simulink model "Rearranged_With_Subsystems"  (R2022b)
settings: Solver=ode15s  StartTime=0.0  StopTime=400  RelTol=1e-3
InitFcn:
  | ManipulatorSetup
  | init_quad_new_leg_raibert_strategy_v2
values from neighbouring files (symbols this model uses):
  body = 'obstacle'+string(i)    [GUIWithNavigation.m]    (also in RunModel.m)
  endx = 18    [EnvironmentData.mat]    (also in Practice data.mat = 15)
  endy = 18    [EnvironmentData.mat]    (also in Practice data.mat = 14)
  floorl = 20    [EnvironmentData.mat]    (also in GUIWithNavigation.m; Practice data.mat; RunModel.m)
  floorw = 20    [EnvironmentData.mat]    (also in GUIWithNavigation.m; Practice data.mat; RunModel.m)
  planner = plannerRRTStar(ss,stateValidator)    [GUIWithNavigation.m]    (also in RunModel.m)
  startx = 3    [EnvironmentData.mat]    (also in Practice data.mat = 2)
  starty = 3    [EnvironmentData.mat]    (also in Practice data.mat = 2)
  tar1Len = 10    [EnvironmentData.mat]    (also in GUIWithNavigation.m = length(target1); Practice data.mat = 13; RunModel.m = length(target1))
  target = [3 4.99844642156 6.95141646815 8.78790598722 9.67257563911 9.70990834754 10.5092252376 9.30187214417 9.05327436398 9.4 9.4 10.8486938703 ... (44 elements, 22x2)]    [EnvironmentData.mat]    (also in GUIWithNavigation.m = cat(1,target1,target2); Practice data.mat = [2 3.44057581018 5.07942513831 5.42542290116 7.21306818311 8; RunModel.m = cat(1,target1,target2))
  tarLen = 22    [EnvironmentData.mat]    (also in RunModel.m = length(target))
undefined symbols (not defined in the file or in its folder): closeFingers, ctrl, Extr_Data_LinkEndHole, grabObjectAngles, grabObjectAngles2, ground, holdFingers, homeAngles, inverseKinematicWeights, l1, l2, m1, m2, openFingers, readyAngles, X, Y, Z
libraries: sm_lib x459, nesl_utility x134, slpidlib x31, fl_ps_legacy_lib x6, robotmaniplib x6, simulink x5, fl_lib x5, Contact_Forces_Lib x4, Parts_Lib x4, sharedtransform x2, dspstat3 x1
(part 15 of 16)

== system Rearranged_With_Subsystems/Quadruped/leg_rr/s_joint_ctrl  ==
  tgt_angle : Inport
  has_ctrl : Inport  Port=2
  PID Controller : slpidlib/PID Controller  Controller=PID  Form=Parallel  TimeDomain=Continuous-time  UseExternalTs=off  SampleTime=-1  IntegratorMethod=Forward Euler  FilterMethod=Forward Euler  ControllerParametersSource=internal  P=ctrl.pos_kp  I=ctrl.pos_ki  UseKiTs=off  D=ctrl.pos_kd  N=100  UseFilter=on  TunerSelectOption=Transfer Function Based (PID Tuner App)  InitialConditionSource=internal  InitialConditionForIntegrator=0  InitialConditionForFilter=0  DifferentiatorICPrevScaledInput=0  ExternalReset=none  TrackingMode=off  Kt=1  LimitOutput=off  SatLimitsSource=internal  UpperSaturationLimit=inf  LowerSaturationLimit=-inf  LinearizeAsGain=on  AntiWindupMode=none  Kb=1  LimitIntegrator=off  UpperIntegratorSaturationLimit=inf  LowerIntegratorSaturationLimit=-inf  POutMin=[]  POutMax=[]  IOutMin=[]  IOutMax=[]  DOutMin=[]  DOutMax=[]  NOutMin=[]  NOutMax=[]  SumOutMin=[]  SumOutMax=[]  SaturationOutMin=[]  SaturationOutMax=[]  PParamMin=[]  PParamMax=[]  IParamMin=[]  IParamMax=[]  DParamMin=[]  DParamMax=[]  NParamMin=[]  NParamMax=[]  KbParamMin=[]  KbParamMax=[]  KtParamMin=[]  KtParamMax=[]  KbOutMin=[]  KbOutMax=[]  KtOutMin=[]  KtOutMax=[]  IntegratorOutMin=[]  IntegratorOutMax=[]  FilterOutMin=[]  FilterOutMax=[]  SumI1OutMin=[]  SumI1OutMax=[]  SumI2OutMin=[]  SumI2OutMax=[]  SumI3OutMin=[]  SumI3OutMax=[]  SumI4OutMin=[]  SumI4OutMax=[]  SumDOutMin=[]  SumDOutMax=[]  DifferentiatorOutMin=[]  DifferentiatorOutMax=[]  FilterDiffOutCoefMin=[]  FilterDiffOutCoefMax=[]  ReciprocalOutMin=[]  ReciprocalOutMax=[]  SumDenOutMin=[]  SumDenOutMax=[]  SumNumOutMin=[]  SumNumOutMax=[]  DivideOutMin=[]  DivideOutMax=[]  UdiffTsProdOutMin=[]  UdiffTsProdOutMax=[]  NTsProdOutMin=[]  NTsProdOutMax=[]  UintegralTsProdOutMin=[]  UintegralTsProdOutMax=[]  UngainTsProdOutMin=[]  UngainTsProdOutMax=[]  ClampingZeroOutDataTypeStr=Inherit: Inherit via back propagation  ClampingZeroOutMin=[]  ClampingZeroOutMax=[]  FilterDenConstantOutDataTypeStr=Inherit: Inherit via back propagation  FilterDenConstantOutMin=[]  FilterDenConstantOutMax=[]  PCopyOutDataTypeStr=Inherit: Inherit via back propagation  PCopyOutMin=[]  PCopyOutMax=[]  NCopyOutDataTypeStr=Inherit: Inherit via back propagation  NCopyOutMin=[]  NCopyOutMax=[]  IntegratorContinuousStateAttributes=''  IntegratorStateMustResolveToSignalObject=off  IntegratorRTWStateStorageClass=Auto  FilterContinuousStateAttributes=''  FilterStateMustResolveToSignalObject=off  FilterRTWStateStorageClass=Auto  ParallelPVariant=InternalParameters  IdealPVariant=Disabled  IVariant=InternalParameters  DVariant=InternalParameters  IntegratorVariant=Continuous  SatVariant=Disabled  AWVariant=Passthrough  PCopyVariant=Disabled  TRVariant=Disabled  FdbkBlocksVariant=Forward  IdealPFdbkVariant=Disabled  SatFdbkVariant=Disabled  DerivativeFilterVariant=ContFilter  NVariant=InternalParameters  NCopyVariant=Disabled  FilterICVariant=InternalICsFilter  IntegratorICVariant=InternalICs  ExternalResetVariant=Disabled  TRSumVariant=Passthrough  SumFdbkVariant=Disabled  SumVariant=Sum_PID  TsampFilterVariant=InternalTs  TsampNgainVariant=Passthrough  TsampIntegralVariant=Passthrough  ExternalSaturationOutDataTypeStr=Inherit: Same as second input
  PID Controller3 : slpidlib/PID Controller  Controller=PID  Form=Parallel  TimeDomain=Continuous-time  UseExternalTs=off  SampleTime=-1  IntegratorMethod=Forward Euler  FilterMethod=Forward Euler  ControllerParametersSource=internal  P=ctrl.vel_kp  I=ctrl.vel_ki  UseKiTs=off  D=ctrl.vel_kd  N=100  UseFilter=on  TunerSelectOption=Transfer Function Based (PID Tuner App)  InitialConditionSource=internal  InitialConditionForIntegrator=0  InitialConditionForFilter=0  DifferentiatorICPrevScaledInput=0  ExternalReset=none  TrackingMode=off  Kt=1  LimitOutput=off  SatLimitsSource=internal  UpperSaturationLimit=inf  LowerSaturationLimit=-inf  LinearizeAsGain=on  AntiWindupMode=none  Kb=1  LimitIntegrator=off  UpperIntegratorSaturationLimit=inf  LowerIntegratorSaturationLimit=-inf  POutMin=[]  POutMax=[]  IOutMin=[]  IOutMax=[]  DOutMin=[]  DOutMax=[]  NOutMin=[]  NOutMax=[]  SumOutMin=[]  SumOutMax=[]  SaturationOutMin=[]  SaturationOutMax=[]  PParamMin=[]  PParamMax=[]  IParamMin=[]  IParamMax=[]  DParamMin=[]  DParamMax=[]  NParamMin=[]  NParamMax=[]  KbParamMin=[]  KbParamMax=[]  KtParamMin=[]  KtParamMax=[]  KbOutMin=[]  KbOutMax=[]  KtOutMin=[]  KtOutMax=[]  IntegratorOutMin=[]  IntegratorOutMax=[]  FilterOutMin=[]  FilterOutMax=[]  SumI1OutMin=[]  SumI1OutMax=[]  SumI2OutMin=[]  SumI2OutMax=[]  SumI3OutMin=[]  SumI3OutMax=[]  SumI4OutMin=[]  SumI4OutMax=[]  SumDOutMin=[]  SumDOutMax=[]  DifferentiatorOutMin=[]  DifferentiatorOutMax=[]  FilterDiffOutCoefMin=[]  FilterDiffOutCoefMax=[]  ReciprocalOutMin=[]  ReciprocalOutMax=[]  SumDenOutMin=[]  SumDenOutMax=[]  SumNumOutMin=[]  SumNumOutMax=[]  DivideOutMin=[]  DivideOutMax=[]  UdiffTsProdOutMin=[]  UdiffTsProdOutMax=[]  NTsProdOutMin=[]  NTsProdOutMax=[]  UintegralTsProdOutMin=[]  UintegralTsProdOutMax=[]  UngainTsProdOutMin=[]  UngainTsProdOutMax=[]  ClampingZeroOutDataTypeStr=Inherit: Inherit via back propagation  ClampingZeroOutMin=[]  ClampingZeroOutMax=[]  FilterDenConstantOutDataTypeStr=Inherit: Inherit via back propagation  FilterDenConstantOutMin=[]  FilterDenConstantOutMax=[]  PCopyOutDataTypeStr=Inherit: Inherit via back propagation  PCopyOutMin=[]  PCopyOutMax=[]  NCopyOutDataTypeStr=Inherit: Inherit via back propagation  NCopyOutMin=[]  NCopyOutMax=[]  IntegratorContinuousStateAttributes=''  IntegratorStateMustResolveToSignalObject=off  IntegratorRTWStateStorageClass=Auto  FilterContinuousStateAttributes=''  FilterStateMustResolveToSignalObject=off  FilterRTWStateStorageClass=Auto  ParallelPVariant=InternalParameters  IdealPVariant=Disabled  IVariant=InternalParameters  DVariant=InternalParameters  IntegratorVariant=Continuous  SatVariant=Disabled  AWVariant=Passthrough  PCopyVariant=Disabled  TRVariant=Disabled  FdbkBlocksVariant=Forward  IdealPFdbkVariant=Disabled  SatFdbkVariant=Disabled  DerivativeFilterVariant=ContFilter  NVariant=InternalParameters  NCopyVariant=Disabled  FilterICVariant=InternalICsFilter  IntegratorICVariant=InternalICs  ExternalResetVariant=Disabled  TRSumVariant=Passthrough  SumFdbkVariant=Disabled  SumVariant=Sum_PID  TsampFilterVariant=InternalTs  TsampNgainVariant=Passthrough  TsampIntegralVariant=Passthrough  ExternalSaturationOutDataTypeStr=Inherit: Same as second input
  PSConv3 : nesl_utility/PS-Simulink Converter  PhysicalDomain=network_engine_domain  SubClassName=ps_output  LeftPortType=input  RightPortType=output  PseudoPeriodic=off  Frequencies=[]  VectorFormat=1-D array  Unit=1  AffineConversion=off
  PSConv4 : nesl_utility/PS-Simulink Converter  PhysicalDomain=network_engine_domain  SubClassName=ps_output  LeftPortType=input  RightPortType=output  PseudoPeriodic=off  Frequencies=[]  VectorFormat=1-D array  Unit=1  AffineConversion=off
  Product : Product
  SPConv : nesl_utility/Simulink-PS Converter  PhysicalDomain=network_engine_domain  SubClassName=ps_input  LeftPortType=input  RightPortType=output  PseudoPeriodic=off  Frequencies=[]  NoiseDistribution=none  NoiseParameters=[]  Unit=1  AffineConversion=off  FilteringAndDerivatives=filter  SimscapeFilterOrder=2  InputFilterTimeConstant=0.001  UdotUserProvided=1
  Sum1 : Sum  Inputs=|+-
  Sum6 : Sum  Inputs=|+-
  curr_angle : PMIOPort  Side=Left
  curr_omega : PMIOPort  Port=2  Side=Left
  torque : PMIOPort  Port=3  Side=Right
  wires:
  tgt_angle/1 -> Sum1/1
  Sum1/1 -> PID Controller/1
  PID Controller/1 -> Sum6/1
  Sum6/1 -> PID Controller3/1
  Product/1 -> SPConv/1
  PSConv3/1 -> Sum1/2
  has_ctrl/1 -> Product/1
  PID Controller3/1 -> Product/2
  PSConv4/1 -> Sum6/2
  connections:
  PSConv3/LConn1 -- curr_angle/RConn1
  SPConv/RConn1 -- torque/RConn1
  curr_omega/RConn1 -- PSConv4/LConn1

== system Rearranged_With_Subsystems/Quadruped/leg_rr/u_joint_ctrl  ==
  tgt_angle : Inport
  has_ctrl : Inport  Port=2
  PID Controller : slpidlib/PID Controller  Controller=PID  Form=Parallel  TimeDomain=Continuous-time  UseExternalTs=off  SampleTime=-1  IntegratorMethod=Forward Euler  FilterMethod=Forward Euler  ControllerParametersSource=internal  P=ctrl.pos_kp  I=ctrl.pos_ki  UseKiTs=off  D=ctrl.pos_kd  N=100  UseFilter=on  TunerSelectOption=Transfer Function Based (PID Tuner App)  InitialConditionSource=internal  InitialConditionForIntegrator=0  InitialConditionForFilter=0  DifferentiatorICPrevScaledInput=0  ExternalReset=none  TrackingMode=off  Kt=1  LimitOutput=off  SatLimitsSource=internal  UpperSaturationLimit=inf  LowerSaturationLimit=-inf  LinearizeAsGain=on  AntiWindupMode=none  Kb=1  LimitIntegrator=off  UpperIntegratorSaturationLimit=inf  LowerIntegratorSaturationLimit=-inf  POutMin=[]  POutMax=[]  IOutMin=[]  IOutMax=[]  DOutMin=[]  DOutMax=[]  NOutMin=[]  NOutMax=[]  SumOutMin=[]  SumOutMax=[]  SaturationOutMin=[]  SaturationOutMax=[]  PParamMin=[]  PParamMax=[]  IParamMin=[]  IParamMax=[]  DParamMin=[]  DParamMax=[]  NParamMin=[]  NParamMax=[]  KbParamMin=[]  KbParamMax=[]  KtParamMin=[]  KtParamMax=[]  KbOutMin=[]  KbOutMax=[]  KtOutMin=[]  KtOutMax=[]  IntegratorOutMin=[]  IntegratorOutMax=[]  FilterOutMin=[]  FilterOutMax=[]  SumI1OutMin=[]  SumI1OutMax=[]  SumI2OutMin=[]  SumI2OutMax=[]  SumI3OutMin=[]  SumI3OutMax=[]  SumI4OutMin=[]  SumI4OutMax=[]  SumDOutMin=[]  SumDOutMax=[]  DifferentiatorOutMin=[]  DifferentiatorOutMax=[]  FilterDiffOutCoefMin=[]  FilterDiffOutCoefMax=[]  ReciprocalOutMin=[]  ReciprocalOutMax=[]  SumDenOutMin=[]  SumDenOutMax=[]  SumNumOutMin=[]  SumNumOutMax=[]  DivideOutMin=[]  DivideOutMax=[]  UdiffTsProdOutMin=[]  UdiffTsProdOutMax=[]  NTsProdOutMin=[]  NTsProdOutMax=[]  UintegralTsProdOutMin=[]  UintegralTsProdOutMax=[]  UngainTsProdOutMin=[]  UngainTsProdOutMax=[]  ClampingZeroOutDataTypeStr=Inherit: Inherit via back propagation  ClampingZeroOutMin=[]  ClampingZeroOutMax=[]  FilterDenConstantOutDataTypeStr=Inherit: Inherit via back propagation  FilterDenConstantOutMin=[]  FilterDenConstantOutMax=[]  PCopyOutDataTypeStr=Inherit: Inherit via back propagation  PCopyOutMin=[]  PCopyOutMax=[]  NCopyOutDataTypeStr=Inherit: Inherit via back propagation  NCopyOutMin=[]  NCopyOutMax=[]  IntegratorContinuousStateAttributes=''  IntegratorStateMustResolveToSignalObject=off  IntegratorRTWStateStorageClass=Auto  FilterContinuousStateAttributes=''  FilterStateMustResolveToSignalObject=off  FilterRTWStateStorageClass=Auto  ParallelPVariant=InternalParameters  IdealPVariant=Disabled  IVariant=InternalParameters  DVariant=InternalParameters  IntegratorVariant=Continuous  SatVariant=Disabled  AWVariant=Passthrough  PCopyVariant=Disabled  TRVariant=Disabled  FdbkBlocksVariant=Forward  IdealPFdbkVariant=Disabled  SatFdbkVariant=Disabled  DerivativeFilterVariant=ContFilter  NVariant=InternalParameters  NCopyVariant=Disabled  FilterICVariant=InternalICsFilter  IntegratorICVariant=InternalICs  ExternalResetVariant=Disabled  TRSumVariant=Passthrough  SumFdbkVariant=Disabled  SumVariant=Sum_PID  TsampFilterVariant=InternalTs  TsampNgainVariant=Passthrough  TsampIntegralVariant=Passthrough  ExternalSaturationOutDataTypeStr=Inherit: Same as second input
  PID Controller3 : slpidlib/PID Controller  Controller=PID  Form=Parallel  TimeDomain=Continuous-time  UseExternalTs=off  SampleTime=-1  IntegratorMethod=Forward Euler  FilterMethod=Forward Euler  ControllerParametersSource=internal  P=ctrl.vel_kp  I=ctrl.vel_ki  UseKiTs=off  D=ctrl.vel_kd  N=100  UseFilter=on  TunerSelectOption=Transfer Function Based (PID Tuner App)  InitialConditionSource=internal  InitialConditionForIntegrator=0  InitialConditionForFilter=0  DifferentiatorICPrevScaledInput=0  ExternalReset=none  TrackingMode=off  Kt=1  LimitOutput=off  SatLimitsSource=internal  UpperSaturationLimit=inf  LowerSaturationLimit=-inf  LinearizeAsGain=on  AntiWindupMode=none  Kb=1  LimitIntegrator=off  UpperIntegratorSaturationLimit=inf  LowerIntegratorSaturationLimit=-inf  POutMin=[]  POutMax=[]  IOutMin=[]  IOutMax=[]  DOutMin=[]  DOutMax=[]  NOutMin=[]  NOutMax=[]  SumOutMin=[]  SumOutMax=[]  SaturationOutMin=[]  SaturationOutMax=[]  PParamMin=[]  PParamMax=[]  IParamMin=[]  IParamMax=[]  DParamMin=[]  DParamMax=[]  NParamMin=[]  NParamMax=[]  KbParamMin=[]  KbParamMax=[]  KtParamMin=[]  KtParamMax=[]  KbOutMin=[]  KbOutMax=[]  KtOutMin=[]  KtOutMax=[]  IntegratorOutMin=[]  IntegratorOutMax=[]  FilterOutMin=[]  FilterOutMax=[]  SumI1OutMin=[]  SumI1OutMax=[]  SumI2OutMin=[]  SumI2OutMax=[]  SumI3OutMin=[]  SumI3OutMax=[]  SumI4OutMin=[]  SumI4OutMax=[]  SumDOutMin=[]  SumDOutMax=[]  DifferentiatorOutMin=[]  DifferentiatorOutMax=[]  FilterDiffOutCoefMin=[]  FilterDiffOutCoefMax=[]  ReciprocalOutMin=[]  ReciprocalOutMax=[]  SumDenOutMin=[]  SumDenOutMax=[]  SumNumOutMin=[]  SumNumOutMax=[]  DivideOutMin=[]  DivideOutMax=[]  UdiffTsProdOutMin=[]  UdiffTsProdOutMax=[]  NTsProdOutMin=[]  NTsProdOutMax=[]  UintegralTsProdOutMin=[]  UintegralTsProdOutMax=[]  UngainTsProdOutMin=[]  UngainTsProdOutMax=[]  ClampingZeroOutDataTypeStr=Inherit: Inherit via back propagation  ClampingZeroOutMin=[]  ClampingZeroOutMax=[]  FilterDenConstantOutDataTypeStr=Inherit: Inherit via back propagation  FilterDenConstantOutMin=[]  FilterDenConstantOutMax=[]  PCopyOutDataTypeStr=Inherit: Inherit via back propagation  PCopyOutMin=[]  PCopyOutMax=[]  NCopyOutDataTypeStr=Inherit: Inherit via back propagation  NCopyOutMin=[]  NCopyOutMax=[]  IntegratorContinuousStateAttributes=''  IntegratorStateMustResolveToSignalObject=off  IntegratorRTWStateStorageClass=Auto  FilterContinuousStateAttributes=''  FilterStateMustResolveToSignalObject=off  FilterRTWStateStorageClass=Auto  ParallelPVariant=InternalParameters  IdealPVariant=Disabled  IVariant=InternalParameters  DVariant=InternalParameters  IntegratorVariant=Continuous  SatVariant=Disabled  AWVariant=Passthrough  PCopyVariant=Disabled  TRVariant=Disabled  FdbkBlocksVariant=Forward  IdealPFdbkVariant=Disabled  SatFdbkVariant=Disabled  DerivativeFilterVariant=ContFilter  NVariant=InternalParameters  NCopyVariant=Disabled  FilterICVariant=InternalICsFilter  IntegratorICVariant=InternalICs  ExternalResetVariant=Disabled  TRSumVariant=Passthrough  SumFdbkVariant=Disabled  SumVariant=Sum_PID  TsampFilterVariant=InternalTs  TsampNgainVariant=Passthrough  TsampIntegralVariant=Passthrough  ExternalSaturationOutDataTypeStr=Inherit: Same as second input
  PSConv3 : nesl_utility/PS-Simulink Converter  PhysicalDomain=network_engine_domain  SubClassName=ps_output  LeftPortType=input  RightPortType=output  PseudoPeriodic=off  Frequencies=[]  VectorFormat=1-D array  Unit=1  AffineConversion=off
  PSConv4 : nesl_utility/PS-Simulink Converter  PhysicalDomain=network_engine_domain  SubClassName=ps_output  LeftPortType=input  RightPortType=output  PseudoPeriodic=off  Frequencies=[]  VectorFormat=1-D array  Unit=1  AffineConversion=off
  Product : Product
  SPConv : nesl_utility/Simulink-PS Converter  PhysicalDomain=network_engine_domain  SubClassName=ps_input  LeftPortType=input  RightPortType=output  PseudoPeriodic=off  Frequencies=[]  NoiseDistribution=none  NoiseParameters=[]  Unit=1  AffineConversion=off  FilteringAndDerivatives=filter  SimscapeFilterOrder=2  InputFilterTimeConstant=0.001  UdotUserProvided=1
  Sum1 : Sum  Inputs=|+-
  Sum6 : Sum  Inputs=|+-
  curr_angle : PMIOPort  Side=Left
  curr_omega : PMIOPort  Port=2  Side=Left
  torque : PMIOPort  Port=3  Side=Right
  wires:
  PSConv4/1 -> Sum6/2
  PID Controller3/1 -> Product/2
  has_ctrl/1 -> Product/1
  PSConv3/1 -> Sum1/2
  Product/1 -> SPConv/1
  Sum6/1 -> PID Controller3/1
  PID Controller/1 -> Sum6/1
  Sum1/1 -> PID Controller/1
  tgt_angle/1 -> Sum1/1
  connections:
  curr_omega/RConn1 -- PSConv4/LConn1
  SPConv/RConn1 -- torque/RConn1
  PSConv3/LConn1 -- curr_angle/RConn1

== system Rearranged_With_Subsystems/Quadruped/leg_rr/upper_leg ==
  note: Geometry Only
  Cap B Left : sm_lib/Body Elements/Extruded Solid  GraphicAmbientColor=[0.15 0.15 0.15 1.0]  BasedOnType=Density  CenterOfMass=[0 0 0]  CenterOfMassUnits=m  GraphicDiffuseColor=[0.2 0.4 0.6]  ExportConvexHullGeometry=off  ExtrusionCrossSection=Extr_Data_LinkEndHole(l1*0.1,l1*0.025,0.05*l1)  ExtrusionCrossSectionUnits=m  Density=0  DensityUnits=kg/m^3  DoExposeReferenceFrame=on  GraphicEmissiveColor=[0.0 0.0 0.0 1.0]  ExportEntireGeometry=off  ExtrusionLength=l1*0.1/3  ExtrusionLengthUnits=m  ExtrusionType=General  SerializedFrames=<Frames/>  MarkerShape=Sphere  MarkerSize=10  GraphicType=FromGeometry  InertiaType=CalculateFromGeometry  Mass=1  MassUnits=kg  MomentsOfInertia=[1 1 1]  MomentsOfInertiaUnits=kg*m^2  PolygonNumSides=3  GraphicOpacity=1.0  PolygonOuterRadius=1  PolygonOuterRadiusUnits=m  ProductsOfInertia=[1 1 1]  ProductsOfInertiaUnits=kg*m^2  GraphicShininess=75  GraphicSpecularColor=[0.5 0.5 0.5 1.0]  GraphicVisPropType=SimpleVisualProperties
  Cap B Right : sm_lib/Body Elements/Extruded Solid  GraphicAmbientColor=[0.15 0.15 0.15 1.0]  BasedOnType=Density  CenterOfMass=[0 0 0]  CenterOfMassUnits=m  GraphicDiffuseColor=[0.2 0.4 0.6]  ExportConvexHullGeometry=off  ExtrusionCrossSection=Extr_Data_LinkEndHole(l1*0.1,l1*0.025,0.05*l1)  ExtrusionCrossSectionUnits=m  Density=0  DensityUnits=kg/m^3  DoExposeReferenceFrame=on  GraphicEmissiveColor=[0.0 0.0 0.0 1.0]  ExportEntireGeometry=off  ExtrusionLength=l1*0.1/3  ExtrusionLengthUnits=m  ExtrusionType=General  SerializedFrames=<Frames/>  MarkerShape=Sphere  MarkerSize=10  GraphicType=FromGeometry  InertiaType=CalculateFromGeometry  Mass=1  MassUnits=kg  MomentsOfInertia=[1 1 1]  MomentsOfInertiaUnits=kg*m^2  PolygonNumSides=3  GraphicOpacity=1.0  PolygonOuterRadius=1  PolygonOuterRadiusUnits=m  ProductsOfInertia=[1 1 1]  ProductsOfInertiaUnits=kg*m^2  GraphicShininess=75  GraphicSpecularColor=[0.5 0.5 0.5 1.0]  GraphicVisPropType=SimpleVisualProperties
  Cap F : sm_lib/Body Elements/Extruded Solid  GraphicAmbientColor=[0.15 0.15 0.15 1.0]  BasedOnType=Density  CenterOfMass=[0 0 0]  CenterOfMassUnits=m  GraphicDiffuseColor=[0.2 0.4 0.6]  ExportConvexHullGeometry=off  ExtrusionCrossSection=Extr_Data_LinkEndHole(l1*0.1,l1*0.025,0.05*l1)  ExtrusionCrossSectionUnits=m  Density=0  DensityUnits=kg/m^3  DoExposeReferenceFrame=on  GraphicEmissiveColor=[0.0 0.0 0.0 1.0]  ExportEntireGeometry=off  ExtrusionLength=l1*0.1  ExtrusionLengthUnits=m  ExtrusionType=General  SerializedFrames=<Frames/>  MarkerShape=Sphere  MarkerSize=10  GraphicType=FromGeometry  InertiaType=CalculateFromGeometry  Mass=1  MassUnits=kg  MomentsOfInertia=[1 1 1]  MomentsOfInertiaUnits=kg*m^2  PolygonNumSides=3  GraphicOpacity=1.0  PolygonOuterRadius=1  PolygonOuterRadiusUnits=m  ProductsOfInertia=[1 1 1]  ProductsOfInertiaUnits=kg*m^2  GraphicShininess=75  GraphicSpecularColor=[0.5 0.5 0.5 1.0]  GraphicVisPropType=SimpleVisualProperties
  Rigid Transform : sm_lib/Frames and Transforms/Rigid Transform  TranslationMethod=StandardAxis  TranslationStandardOffset=0.1*l1/3  TranslationLengthUnit=m  TranslationStandardAxis=+Z  TranslationCartesianOffset=[0 0 0]  TranslationROffset=0  TranslationROffsetUnits=m  TranslationZOffset=0  TranslationZOffsetUnits=m  TranslationThetaOffset=0  TranslationThetaOffsetUnits=deg  RotationMethod=StandardAxis  RotationAngleUnits=deg  RotationStandardAxis=+Z  RotationAngle=-90  RotationArbitraryAxis=[0 0 1]  FollAlignAxisA=+X  BaseAlignAxisA=+Y  FollAlignAxisB=+Y  BaseAlignAxisB=+Z  RotationSequenceAxes=FollowerAxes  RotationSequence=XYX  RotationSequenceAngles=[0 0 0]  RotationSequenceAnglesUnits=deg  RotationMatrix=[1 0 0; 0 1 0; 0 0 1]  Quaternion=[1 0 0 0]
  Transform B : sm_lib/Frames and Transforms/Rigid Transform  TranslationMethod=StandardAxis  TranslationStandardOffset=body.upper_length/2  TranslationLengthUnit=m  TranslationStandardAxis=+Y  TranslationCartesianOffset=[0 0 0]  TranslationROffset=0  TranslationROffsetUnits=m  TranslationZOffset=0  TranslationZOffsetUnits=m  TranslationThetaOffset=0  TranslationThetaOffsetUnits=deg  RotationMethod=StandardAxis  RotationAngleUnits=deg  RotationStandardAxis=+Z  RotationAngle=180  RotationArbitraryAxis=[0 0 1]  FollAlignAxisA=+X  BaseAlignAxisA=+Y  FollAlignAxisB=+Y  BaseAlignAxisB=+Z  RotationSequenceAxes=FollowerAxes  RotationSequence=XYX  RotationSequenceAngles=[0 0 0]  RotationSequenceAnglesUnits=deg  RotationMatrix=[1 0 0; 0 1 0; 0 0 1]  Quaternion=[1 0 0 0]
  Transform Cap F : sm_lib/Frames and Transforms/Rigid Transform  TranslationMethod=None  TranslationStandardOffset=0  TranslationLengthUnit=m  TranslationStandardAxis=+Z  TranslationCartesianOffset=[0 0 0]  TranslationROffset=0  TranslationROffsetUnits=m  TranslationZOffset=0  TranslationZOffsetUnits=m  TranslationThetaOffset=0  TranslationThetaOffsetUnits=deg  RotationMethod=StandardAxis  RotationAngleUnits=deg  RotationStandardAxis=+Z  RotationAngle=90  RotationArbitraryAxis=[0 0 1]  FollAlignAxisA=+X  BaseAlignAxisA=+Y  FollAlignAxisB=+Y  BaseAlignAxisB=+Z  RotationSequenceAxes=FollowerAxes  RotationSequence=XYX  RotationSequenceAngles=[0 0 0]  RotationSequenceAnglesUnits=deg  RotationMatrix=[1 0 0; 0 1 0; 0 0 1]  Quaternion=[1 0 0 0]
  Transform F : sm_lib/Frames and Transforms/Rigid Transform  TranslationMethod=None  TranslationStandardOffset=l1/2  TranslationLengthUnit=m  TranslationStandardAxis=+Y  TranslationCartesianOffset=[0 0 0]  TranslationROffset=0  TranslationROffsetUnits=m  TranslationZOffset=0  TranslationZOffsetUnits=m  TranslationThetaOffset=0  TranslationThetaOffsetUnits=deg  RotationMethod=StandardAxis  RotationAngleUnits=deg  RotationStandardAxis=+Z  RotationAngle=180  RotationArbitraryAxis=[0 0 1]  FollAlignAxisA=+X  BaseAlignAxisA=+Y  FollAlignAxisB=+Y  BaseAlignAxisB=+Z  RotationSequenceAxes=FollowerAxes  RotationSequence=XYX  RotationSequenceAngles=[0 0 0]  RotationSequenceAnglesUnits=deg  RotationMatrix=[1 0 0; 0 1 0; 0 0 1]  Quaternion=[1 0 0 0]
  Transform R : sm_lib/Frames and Transforms/Rigid Transform  TranslationMethod=StandardAxis  TranslationStandardOffset=body.upper_length/2  TranslationLengthUnit=m  TranslationStandardAxis=+Y  TranslationCartesianOffset=[0 0 0]  TranslationROffset=0  TranslationROffsetUnits=m  TranslationZOffset=0  TranslationZOffsetUnits=m  TranslationThetaOffset=0  TranslationThetaOffsetUnits=deg  RotationMethod=None  RotationAngleUnits=deg  RotationStandardAxis=+Z  RotationAngle=180  RotationArbitraryAxis=[0 0 1]  FollAlignAxisA=+X  BaseAlignAxisA=+Y  FollAlignAxisB=+Y  BaseAlignAxisB=+Z  RotationSequenceAxes=FollowerAxes  RotationSequence=XYX  RotationSequenceAngles=[0 0 0]  RotationSequenceAnglesUnits=deg  RotationMatrix=[1 0 0; 0 1 0; 0 0 1]  Quaternion=[1 0 0 0]
  "Transform Stem " : sm_lib/Frames and Transforms/Rigid Transform  TranslationMethod=StandardAxis  TranslationStandardOffset=-0.1*l1/3  TranslationLengthUnit=m  TranslationStandardAxis=+Z  TranslationCartesianOffset=[0 0 0]  TranslationROffset=0  TranslationROffsetUnits=m  TranslationZOffset=0  TranslationZOffsetUnits=m  TranslationThetaOffset=0  TranslationThetaOffsetUnits=deg  RotationMethod=StandardAxis  RotationAngleUnits=deg  RotationStandardAxis=+Z  RotationAngle=-90  RotationArbitraryAxis=[0 0 1]  FollAlignAxisA=+X  BaseAlignAxisA=+Y  FollAlignAxisB=+Y  BaseAlignAxisB=+Z  RotationSequenceAxes=FollowerAxes  RotationSequence=XYX  RotationSequenceAngles=[0 0 0]  RotationSequenceAnglesUnits=deg  RotationMatrix=[1 0 0; 0 1 0; 0 0 1]  Quaternion=[1 0 0 0]
  Upper Leg : sm_lib/Body Elements/Brick Solid  GraphicAmbientColor=[0.15 0.15 0.15 1.0]  BasedOnType=Density  BrickDimensions=[0.1*l1 body.upper_length-(l1*0.2) 0.1*l1]  BrickDimensionUnits=m  CenterOfMass=[0 0 0]  CenterOfMassUnits=m  GraphicDiffuseColor=[0.2 0.4 0.6]  Density=leg_density  DensityUnits=kg/m^3  DoExposeReferenceFrame=on  GraphicEmissiveColor=[0.0 0.0 0.0 1.0]  ExportEntireGeometry=off  SerializedFrames=<Frames><Frame><Id>Frame1</Id><Value><Name>B</Name><Origin><Source>GeometricFeature</Source><FeatureName>-y surface</FeatureName></Origin><PrimaryAxis><DefinedDirection>+Z</DefinedDirection><Source>ReferenceFrame</Source><SourceDirection>+Z</SourceDirection><FeatureName></FeatureName></PrimaryAxis><SecondaryAxis><DefinedDirection>+X</DefinedDirection><Source>ReferenceFrame</Source><SourceDirection>+X</SourceDirection><FeatureName></FeatureName></SecondaryAxis></Value></Frame><Frame><Id>Frame2</Id><Value><Name>F</Name><Origin><Source>GeometricFeature</Source><FeatureName>+y surface</FeatureName></Origin><PrimaryAxis><DefinedDirection>+Z</DefinedDirection><Source>ReferenceFrame</Source><SourceDirection>+Z</SourceDirection><FeatureName></FeatureName></PrimaryAxis><SecondaryAxis><DefinedDirection>+X</DefinedDirection><Source>ReferenceFrame</Source><SourceDirection>+X</SourceDirection><FeatureName></FeatureName></SecondaryAxis></Value></Frame></Frames>  MarkerShape=Sphere  MarkerSize=10  GraphicType=FromGeometry  InertiaType=CalculateFromGeometry  Mass=m1*l1  MassUnits=kg  MomentsOfInertia=[1 1 1]*(1/12)*m1*l1*l1^2  MomentsOfInertiaUnits=kg*m^2  GraphicOpacity=1.0  ProductsOfInertia=[1 1 1]*0  ProductsOfInertiaUnits=kg*m^2  GraphicShininess=75  GraphicSpecularColor=[0.5 0.5 0.5 1.0]  GraphicVisPropType=SimpleVisualProperties
  joint_upper : PMIOPort  Side=Right
  joint_knee : PMIOPort  Port=2  Side=Left
  connections:
  Transform Cap F/LConn1 -- Upper Leg/LConn2
  "Transform Stem "/RConn1 -- Cap B Left/RConn1
  Upper Leg/LConn1 -- "Transform Stem "/LConn1 -- Rigid Transform/LConn1
  Cap F/RConn1 -- Transform Cap F/RConn1
  Cap B Right/RConn1 -- Rigid Transform/RConn1
  Transform B/LConn1 -- Transform R/RConn1 -- Upper Leg/RConn1
  Transform B/RConn1 -- joint_upper/RConn1
  joint_knee/RConn1 -- Transform F/LConn1
  Transform F/RConn1 -- Transform R/LConn1

== system Rearranged_With_Subsystems/Controller/Subsystem/Path follower/If Action Subsystem ==
  In1 : Inport
  Action Port : ActionPort  ActionPortLabel=if(u1 <= 0)
  Out1 : Outport
  wires:
  In1/1 -> Out1/1

== system Rearranged_With_Subsystems/Controller/Subsystem/Path follower/If Action Subsystem1 ==
  In1 : Inport
  Action Port : ActionPort  ActionPortLabel=else
  Out1 : Outport
  wires:
  In1/1 -> Out1/1

== system Rearranged_With_Subsystems/Manipulator/Subsystem1/Subsystem7/Subsystem ==
  timeValues : Inport
  angleRange : Inport  Port=2
  currentTime : Inport  Port=3
  1-D Lookup Table : Lookup_n-D  NumberOfTableDimensions=1  BreakpointsForDimension1Source=Input port  BreakpointsForDimension1=[-5:5]  TableSource=Input port  Table=tanh([-5:5])  InternalRulePriority=Speed  RndMeth=Simplest
      settings: InputPortMap=u0,p221,p5
  Display : Display
  anglePosition : Outport
  wires:
  timeValues/1 -> 1-D Lookup Table/3
  1-D Lookup Table/1 -> anglePosition/1
  currentTime/1 -> 1-D Lookup Table/1
  angleRange/1 -> 1-D Lookup Table/2, Display/1

== system Rearranged_With_Subsystems/Manipulator/Subsystem1/Subsystem7/Subsystem1 ==
  timeValues : Inport
  angleRange : Inport  Port=2
  currentTime : Inport  Port=3
  1-D Lookup Table : Lookup_n-D  NumberOfTableDimensions=1  BreakpointsForDimension1Source=Input port  BreakpointsForDimension1=[-5:5]  TableSource=Input port  Table=tanh([-5:5])  InternalRulePriority=Speed  RndMeth=Simplest
      settings: InputPortMap=u0,p221,p5
  anglePosition : Outport
  wires:
  timeValues/1 -> 1-D Lookup Table/3
  1-D Lookup Table/1 -> anglePosition/1
  currentTime/1 -> 1-D Lookup Table/1
  angleRange/1 -> 1-D Lookup Table/2

== system Rearranged_With_Subsystems/Manipulator/Subsystem1/Subsystem7/Subsystem2 ==
  timeValues : Inport
  angleRange : Inport  Port=2
  currentTime : Inport  Port=3
  1-D Lookup Table : Lookup_n-D  NumberOfTableDimensions=1  BreakpointsForDimension1Source=Input port  BreakpointsForDimension1=[-5:5]  TableSource=Input port  Table=tanh([-5:5])  InternalRulePriority=Speed  RndMeth=Simplest
      settings: InputPortMap=u0,p221,p5
  anglePosition : Outport
  wires:
  timeValues/1 -> 1-D Lookup Table/3
  1-D Lookup Table/1 -> anglePosition/1
  currentTime/1 -> 1-D Lookup Table/1
  angleRange/1 -> 1-D Lookup Table/2

== system Rearranged_With_Subsystems/Manipulator/Subsystem1/Subsystem7/Subsystem3 ==
  timeValues : Inport
  angleRange : Inport  Port=2
  currentTime : Inport  Port=3
  1-D Lookup Table : Lookup_n-D  NumberOfTableDimensions=1  BreakpointsForDimension1Source=Input port  BreakpointsForDimension1=[-5:5]  TableSource=Input port  Table=tanh([-5:5])  InternalRulePriority=Speed  RndMeth=Simplest
      settings: InputPortMap=u0,p221,p5
  anglePosition : Outport
  wires:
  timeValues/1 -> 1-D Lookup Table/3
  1-D Lookup Table/1 -> anglePosition/1
  currentTime/1 -> 1-D Lookup Table/1
  angleRange/1 -> 1-D Lookup Table/2

== system Rearranged_With_Subsystems/Manipulator/Subsystem1/Subsystem7/Subsystem4 ==
  timeValues : Inport
  angleRange : Inport  Port=2
  currentTime : Inport  Port=3
  1-D Lookup Table : Lookup_n-D  NumberOfTableDimensions=1  BreakpointsForDimension1Source=Input port  BreakpointsForDimension1=[-5:5]  TableSource=Input port  Table=tanh([-5:5])  InternalRulePriority=Speed  RndMeth=Simplest
      settings: InputPortMap=u0,p221,p5
  anglePosition : Outport
  wires:
  timeValues/1 -> 1-D Lookup Table/3
  1-D Lookup Table/1 -> anglePosition/1
  currentTime/1 -> 1-D Lookup Table/1
  angleRange/1 -> 1-D Lookup Table/2

== system Rearranged_With_Subsystems/Manipulator/Subsystem1/Subsystem7/Subsystem5 ==
  timeValues : Inport
  angleRange : Inport  Port=2
  currentTime : Inport  Port=3
  1-D Lookup Table : Lookup_n-D  NumberOfTableDimensions=1  BreakpointsForDimension1Source=Input port  BreakpointsForDimension1=[-5:5]  TableSource=Input port  Table=tanh([-5:5])  InternalRulePriority=Speed  RndMeth=Simplest
      settings: InputPortMap=u0,p221,p5
  anglePosition : Outport
  wires:
  timeValues/1 -> 1-D Lookup Table/3
  1-D Lookup Table/1 -> anglePosition/1
  currentTime/1 -> 1-D Lookup Table/1
  angleRange/1 -> 1-D Lookup Table/2

== system Rearranged_With_Subsystems/Manipulator/Subsystem1/Subsystem7/Subsystem6 ==
  timeValues : Inport
  angleRange : Inport  Port=2
  currentTime : Inport  Port=3
  1-D Lookup Table : Lookup_n-D  NumberOfTableDimensions=1  BreakpointsForDimension1Source=Input port  BreakpointsForDimension1=[-5:5]  TableSource=Input port  Table=tanh([-5:5])  InternalRulePriority=Speed  RndMeth=Simplest
      settings: InputPortMap=u0,p221,p5
  anglePosition : Outport
  wires:
  timeValues/1 -> 1-D Lookup Table/3
  1-D Lookup Table/1 -> anglePosition/1
  currentTime/1 -> 1-D Lookup Table/1
  angleRange/1 -> 1-D Lookup Table/2

== matlab function Rearranged_With_Subsystems/Controller/QuadCtrl ==
  settings: updateMethod=DISCRETE
  data: fl_ang input; tgt_ctrl_fl output; fr_ang input; rl_ang input; rr_ang input; contact_state input; body_R input; sensing_info input; tgt_ctrl_fr output; tgt_ctrl_rl output; tgt_ctrl_rr output; t input; body parameter; planner parameter; mode input; ctrl_state output; debug output; next_state input
function [tgt_ctrl_fl,tgt_ctrl_fr,tgt_ctrl_rl,tgt_ctrl_rr, ctrl_state, debug] = ...
    controller(fl_ang, fr_ang, rl_ang, rr_ang, ...
    contact_state, body_R, sensing_info, t, body, planner, mode, next_state)

%unpack sensing_info
body_vx = sensing_info(4);
body_vy = sensing_info(5);

% distance from center of mass to shoulder
fl_offset = [body.shoulder_distance;body.y_length/2+body.shoulder_size/2;0];
fr_offset = [body.shoulder_distance;-body.y_length/2-body.shoulder_size/2;0];
rl_offset = [-body.shoulder_distance;body.y_length/2+body.shoulder_size/2;0];
rr_offset = [-body.shoulder_distance;-body.y_length/2-body.shoulder_size/2;0];

%decide state and state transition helpers
persistent state;
persistent timer;
persistent timer2;
if isempty(state)
    state = 0;
end
if isempty(timer)
    timer = 0;
end
if isempty(timer2)
    timer2 = 0;
end

% init variables
           % fl fr rl rr
has_u_ctrl = [1 1 1 1];
normal_virtual_leg1 = [0;0;planner.stand_height];
normal_virtual_leg2 = [0;0;planner.stand_height];
move_fl_end_effector = normal_virtual_leg1;
move_rr_end_effector = normal_virtual_leg1;
move_fr_end_effector = normal_virtual_leg2;
move_rl_end_effector = normal_virtual_leg2;

% turning on spot mechanic
isTurning = mode == 2 || mode == 3;
%{
if isTurning
    leg_a_coef = 1; % -1/3
    leg_b_coef = 1;
else
    leg_a_coef = 1;
    leg_b_coef = 1;
end
%}
leg_a_coef = 1;
leg_b_coef = 1;

% state machine

if state == 0 % standby state
    % in this state, just do nothing, but use time to make sure that all
    % feet stands on the ground

    if contact_state(1) == 1 && contact_state(2) == 1 && contact_state(3) == 1 && contact_state(4) == 1
        %all foot on ground
        if abs(body_vx) < planner.state0_vel_thres 
            timer = timer + 1;
        else
            timer = 0;
        end
        if timer > planner.state0_trans_thres 
            state = 1;
            timer = 0;
        end
    end
elseif state == 1 % swing whole body to get a inital velocity
    timer2 = timer2 + 1;
    move_theta = planner.state0_swing_ang*sin(2*pi/planner.state0_swing_T*timer2);
    move_leg_Rx = [cos(move_theta) 0 sin(move_theta);
        0 1 0;
        -sin(move_theta) 0 cos(move_theta)];
    tgt_virtual_leg1_b = move_leg_Rx*normal_virtual_leg1;
    tgt_virtual_leg2_b = move_leg_Rx*normal_virtual_leg2;
    move_fl_end_effector = tgt_virtual_leg1_b;
    move_rr_end_effector = tgt_virtual_leg1_b;
    move_fr_end_effector = tgt_virtual_leg2_b;
    move_rl_end_effector = tgt_virtual_leg2_b;
        
    if body_vx > planner.state12_trans_speed
        timer = timer + 1;
    else
        timer = 0;
    end
    if timer > 40  %(keep a velocity larger than 0.2 for 0.1s)
        state = next_state;
        timer = 0;
        timer2 = 0;
    end

elseif state == 2 % stance virtual leg1, swing virtual leg2
    timer2 = timer2 + 1;
    if timer2 > planner.leg_swing_time %(0.5s finish movement)
        timer2 = planner.leg_swing_time;
    end
    % stance leg no u control but need to balance the body
               % fl fr rl rr
    has_u_ctrl = [0 1 1 0];
    t = timer2/planner.leg_swing_time;
%     stance_length_coeff = 0.95+0.05*(timer2/planner.leg_swing_time);
    stance_length_coeff = 0.2*t^2 - 0.2*t + 1;
    tgt_virtual_leg1_b = stance_length_coeff*normal_virtual_leg1;
    move_fl_end_effector = tgt_virtual_leg1_b;
    move_rr_end_effector = tgt_virtual_leg1_b;
    
    
    % swing leg must consider body angle 
%     move_theta = -11/180*pi*(t);
    length_coeff = 0.8*t^2-0.8*t+1;
    % move leg in x direction
    move_theta = get_move_angle(length_coeff*normal_virtual_leg2,body_vx, planner.tgt_body_vx, planner);
    
    move_leg_Rx = [cos(move_theta) 0 sin(move_theta);
        0 1 0;
        -sin(move_theta) 0 cos(move_theta)];
    move_leg_Rx2 = [cos(move_theta) 0 sin(move_theta);
        0 1 0;
        -sin(move_theta) 0 cos(move_theta)];
    tgt_virtual_leg2_a = length_coeff*move_leg_Rx2*normal_virtual_leg2;
    tgt_virtual_leg2_b = length_coeff*move_leg_Rx*normal_virtual_leg2;
    
    % move leg in y direction
    sagittal_angle = get_sagittal_angle(tgt_virtual_leg2_b,body_R, body_vy, planner);
    move_leg_Ry =[1 0 0;
                 0 cos(sagittal_angle) -sin(sagittal_angle);
                 0 sin(sagittal_angle) cos(sagittal_angle)];
    tgt_virtual_leg2_b = move_leg_Ry*tgt_virtual_leg2_b;
    tgt_virtual_leg2_a = move_leg_Ry*tgt_virtual_leg2_a;
    
    
    move_fr_end_effector = body_R'*(tgt_virtual_leg2_b+fr_offset)-fr_offset;
    if norm(move_fr_end_effector) > body.max_stretch
        move_fr_end_effector = move_fr_end_effector/norm(move_fr_end_effector)*body.max_stretch;
    end
    move_rl_end_effector = body_R'*(tgt_virtual_leg2_a+rl_offset)-rl_offset;
    if norm(move_rl_end_effector) > body.max_stretch
        move_rl_end_effector = move_rl_end_effector/norm(move_rl_end_effector)*body.max_stretch;
    end
    
    % state transition
%     if timer2 == planner.leg_swing_time
    if timer2 > 0.5*planner.leg_swing_time && contact_state(2) == 1 && contact_state(3) == 1
        timer = timer + 1;
    else
        timer = 0;
    end
    if timer > 5   % to be determined
        state = next_state;
        timer = 0;
        timer2 = 0;
    end
    
elseif state == 3 % swing virtual leg1, stance virtual leg2
    timer2 = timer2 + 1;
    if timer2 > planner.leg_swing_time %(0.5s finish movement)
        timer2 = planner.leg_swing_time;
    end
    % stance leg no u control but need to balance the body
               % fl fr rl rr
    has_u_ctrl = [1 0 0 1];
%     stance_length_coeff = 0.95+0.05*(timer2/planner.leg_swing_time);
    t = timer2/planner.leg_swing_time;
    stance_length_coeff = 0.2*t^2 - 0.2*t + 1;
    tgt_virtual_leg2_b = stance_length_coeff*normal_virtual_leg2;
    move_fr_end_effector = tgt_virtual_leg2_b;
    move_rl_end_effector = tgt_virtual_leg2_b;
    
    % swing leg must consider body angle 
    % theta is a function of forward velocity 
%     move_theta = -11/180*pi*(t);
    length_coeff = 0.8*t^2-0.8*t+1;
    move_theta = get_move_angle(length_coeff*normal_virtual_leg1,body_vx, planner.tgt_body_vx, planner);
    move_leg_Rx = [cos(move_theta*(1-2*isTurning)) 0 sin(move_theta*(1-2*isTurning));
        0 1 0;
        -sin(move_theta*(1-2*isTurning)) 0 cos(move_theta*(1-2*isTurning))];
    move_leg_Rx2 = [cos(move_theta*(1-2*isTurning)) 0 sin(move_theta*(1-2*isTurning));
        0 1 0;
        -sin(move_theta*(1-2*isTurning)) 0 cos(move_theta*(1-2*isTurning))];
    tgt_virtual_leg1_a = length_coeff*move_leg_Rx2*normal_virtual_leg1;
    tgt_virtual_leg1_b = length_coeff*move_leg_Rx*normal_virtual_leg1;
    
    % move leg in y direction
    sagittal_angle = get_sagittal_angle(tgt_virtual_leg1_b,body_R, body_vy, planner);
    move_leg_Ry =[1 0 0;
                 0 cos(sagittal_angle) -sin(sagittal_angle);
                 0 sin(sagittal_angle) cos(sagittal_angle)];
    tgt_virtual_leg1_b = move_leg_Ry*tgt_virtual_leg1_b;
    tgt_virtual_leg1_a = move_leg_Ry*tgt_virtual_leg1_a;
    
    move_fl_end_effector = body_R'*(tgt_virtual_leg1_b+fl_offset)-fl_offset;
    if norm(move_fl_end_effector) > body.max_stretch
        move_fl_end_effector = move_fl_end_effector/norm(move_fl_end_effector)*body.max_stretch;
    end
    move_rr_end_effector = body_R'*(tgt_virtual_leg1_a+rr_offset)-rr_offset;
    if norm(move_rr_end_effector) > body.max_stretch
        move_rr_end_effector = move_rr_end_effector/norm(move_rr_end_effector)*body.max_stretch;
    end
    
    % state transition
%     if timer2 == planner.leg_swing_time
    if timer2 > 0.5*planner.leg_swing_time && contact_state(1) == 1 && contact_state(4) == 1
        timer = timer + 1;
    else
        timer = 0;
    end
    if timer > 5   % to be determined
        state = next_state;
        timer = 0;
        timer2 = 0;
    end
elseif state == 4 % stabalisation
    timer2 = timer2 + 1;
    move_theta = planner.state0_swing_ang*sin(2*pi/planner.state0_swing_T*timer2);
    move_leg_Rx = [cos(move_theta) 0 sin(move_theta);
        0 1 0;
        -sin(move_theta) 0 cos(move_theta)];
    tgt_virtual_leg1_b = move_leg_Rx*normal_virtual_leg1;
    tgt_virtual_leg2_b = move_leg_Rx*normal_virtual_leg2;
    move_fl_end_effector = tgt_virtual_leg1_b;
    move_rr_end_effector = tgt_virtual_leg1_b;
    move_fr_end_effector = tgt_virtual_leg2_b;
    move_rl_end_effector = tgt_virtual_leg2_b;
        
    timer = timer + 1;
    if timer > 40  %(keep a velocity larger than 0.2 for 0.1s)
        state = next_state;
        timer = 0;
        timer2 = 0;
    end
end

%% fl to joint
[inv_s,inv_u,inv_k] = inverse_kinematics(move_fl_end_effector, body);
fl_tgt_ang_s = inv_s; 
fl_tgt_ang_u = inv_u;       
fl_tgt_ang_k = inv_k; 
tgt_ctrl_fl = [fl_tgt_ang_s;fl_tgt_ang_u;fl_tgt_ang_k;has_u_ctrl(1)];

%% fr to joint
[inv_s,inv_u,inv_k] = inverse_kinematics(move_fr_end_effector, body);
fr_tgt_ang_s = inv_s;
fr_tgt_ang_u = inv_u;
fr_tgt_ang_k = inv_k;
tgt_ctrl_fr = [fr_tgt_ang_s;fr_tgt_ang_u;fr_tgt_ang_k;has_u_ctrl(2)];

%% rl to joint
[inv_s,inv_u,inv_k] = inverse_kinematics(move_rl_end_effector, body);
rl_tgt_ang_s = inv_s;
rl_tgt_ang_u = inv_u;
rl_tgt_ang_k = inv_k;
tgt_ctrl_rl = [rl_tgt_ang_s;rl_tgt_ang_u;rl_tgt_ang_k;has_u_ctrl(3)];

%% rr to joint
[inv_s,inv_u,inv_k] = inverse_kinematics(move_rr_end_effector, body);
rr_tgt_ang_s = inv_s;
rr_tgt_ang_u = inv_u;
rr_tgt_ang_k = inv_k; 
tgt_ctrl_rr = [rr_tgt_ang_s;rr_tgt_ang_u;rr_tgt_ang_k;has_u_ctrl(4)];

ctrl_state = state;
debug = timer;

end

function move_angle = get_move_angle(virtual_leg,body_vx, tgt_body_vx, planner)

    distance = body_vx* planner.Ts/2 + planner.Kv*(tgt_body_vx-body_vx);
    
    if distance > 0.5*norm(virtual_leg)
        distance = 0.5*norm(virtual_leg);
    elseif distance < -0.5*norm(virtual_leg)
        distance = -0.5*norm(virtual_leg);
    end
    
    move_angle = asin(distance/norm(virtual_leg));
    if move_angle > 20/180*pi
        move_angle = 20/180*pi;
    elseif move_angle < -20/180*pi
        move_angle = -20/180*pi;
    end
    
end

function move_angle = get_sagittal_angle(virtual_leg,body_R, body_vy, planner)

    distance = body_vy* planner.y_Ts/2 + planner.y_Kv*(0-body_vy);  

    if distance > 0.5*norm(virtual_leg)
        distance = 0.5*norm(virtual_leg);
    elseif distance < -0.5*norm(virtual_leg)
        distance = -0.5*norm(virtual_leg);
    end
    
    move_angle = asin(distance/norm(virtual_leg));
    if move_angle > 20/180*pi
        move_angle = 20/180*pi;
    elseif move_angle < -20/180*pi
        move_angle = -20/180*pi;
    end
    
end

== stateflow chart Rearranged_With_Subsystems/Controller/High Level Mode Stateflow ==
  state ResetPos
    mode=0;
    ManipTask=1;
  state Stationary
    mode=0;
    ManipTask=0;
  state Turning_Right
    mode=2;
  state Walking
    mode=1;
  state Turning_Left
    mode=3;
  Turning_Right -> ResetPos [order 2] : [resetPos==1]{pos_index=pos_index+2}
  Stationary -> ResetPos [order 2] : [resetPos==1]{pos_index=pos_index+2}
  ResetPos -> Stationary : [manipState==5]
  Walking -> ResetPos [order 4] : [resetPos==1]{pos_index=pos_index+2}
  Turning_Left -> ResetPos [order 2] : [resetPos==1]{pos_index=pos_index+2}
  (default) -> Stationary : {pos_index =2 }
  Turning_Left -> Stationary [order 1] : [delta_theta < ang_threshold]
  Turning_Right -> Stationary [order 1] : [delta_theta > -ang_threshold]
  Stationary -> Walking [order 1] : [~target_reached]
  Walking -> Stationary [order 3] : [target_reached]
      | {pos_index = pos_index + 1}
  Walking -> Turning_Right [order 2] : [delta_theta < -ang_threshold]
  Walking -> Turning_Left [order 1] : [delta_theta > ang_threshold]
  data: pos_index output =0; mode output =0; target_reached input; delta_theta input; ang_threshold local =0.2; resetPos input; ManipTask output; manipState input

== stateflow chart Rearranged_With_Subsystems/Controller/Chart ==
  state PathFollowing
    resetPos=0;
  state ManipulatorTask
    resetPos=1;
  (default) -> PathFollowing
  PathFollowing -> ManipulatorTask : [pos_index==tar1Len]
  ManipulatorTask -> PathFollowing : [manipState==5]
  data: pos_index input; tar1Len input; resetPos output; manipState input

== matlab function Rearranged_With_Subsystems/Manipulator/Ball Tracking and Handling/MATLAB Function1 ==
  data: objectTransform output; x input; y input; z input; aboveObjectTransform output
function [objectTransform,aboveObjectTransform] = fcn(x,y,z)
rotTransform=[1 0 0;0 -1 0;0 0 -1];
F=rotTransform;
xline=F(1,:);
yline=F(2,:);
zline=F(3,:);
objectTransform = [ xline x;yline y;zline z+0.02;0 0 0 1];
aboveObjectTransform = [xline x;yline y;zline z+0.1;0 0 0 1];

== matlab function Rearranged_With_Subsystems/Manipulator1/MATLAB Function ==
  settings: updateMethod=DISCRETE
  data: quadrupedInPosition input; errorVals input; contactForces input; state input; y output; readyAngles input; grabObjectAngles2 input; grabObjectAngles input; openFingers input; closeFingers input; holdFingers input; stateOut output; objectPosition input; aboveObjectPosition input
function [y,stateOut] = fcn(quadrupedInPosition,errorVals,contactForces,state,readyAngles,grabObjectAngles2,grabObjectAngles,openFingers,closeFingers,holdFingers,objectPosition,aboveObjectPosition)

if quadrupedInPosition == 1
    state = int16(state);

    switch state
        case 0
            y = [readyAngles;openFingers];
        case 1

            y = [aboveObjectPosition;openFingers];
        case 2
            y = [objectPosition;openFingers];
        case 3
            y = [objectPosition;closeFingers];
        case 4
            y = [aboveObjectPosition;closeFingers];
        case 5
            y = [readyAngles;closeFingers];
        otherwise
            y = zeros(13,1);
    end
    
    if state == 0 && min(errorVals) >= -0.01 && max(errorVals) <=0.01
        
        stateOut = 1;
        tic;
    elseif state == 1 && min(errorVals) >= -0.01 && max(errorVals) <=0.01 && toc >= 4
        stateOut = 2;
        tic;
    elseif state == 2 && min(errorVals) >= -0.01 && max(errorVals) <=0.01 && toc >= 0.5
        stateOut = 3;
        tic;
    elseif state == 3 && min(contactForces) >= 0.5 && toc >= 1
        toc;
        stateOut = 4;
        tic;
    elseif state == 4 && min(errorVals) >= -0.01 && max(errorVals) <=0.01 && toc >= 10
        stateOut = 5;
    elseif state == 5 && min(errorVals) >= -0.01 && max(errorVals) <=0.01
        stateOut = 5;
    else
        stateOut = double(state);
    end
else
    y = [readyAngles;openFingers];
    stateOut = 0;
end

== matlab function Rearranged_With_Subsystems/Manipulator1/MATLAB Function1 ==
  data: R input; objectTransform output; x input; y input; z input; aboveObjectTransform output
function [objectTransform,aboveObjectTransform] = fcn(R,x,y,z)

objectTransform = [1 0 0 x;0 -1 0 y;0 0 -1 z+0.02;0 0 0 1];
aboveObjectTransform = [1 0 0 x;0 -1 0 y;0 0 -1 z+0.1;0 0 0 1];

== matlab function Rearranged_With_Subsystems/Manipulator/End Tracking and handling/MATLAB Function1 ==
  data: objectTransform output; x input; y input; z input; aboveObjectTransform output
function [objectTransform,aboveObjectTransform] = fcn(x,y,z)
rotTransform=[1 0 0;0 -1 0;0 0 -1];
F=rotTransform;
xline=F(1,:);
yline=F(2,:);
zline=F(3,:);
objectTransform = [ xline x;yline y;zline z+0.02;0 0 0 1];
aboveObjectTransform = [xline x;yline y;zline z+0.1;0 0 0 1];
